simulink model "Lab2_EEN155_BUCK_2023"  (R2022b)
settings: Solver=VariableStepAuto  StartTime=0.0  StopTime=0.5  RelTol=1e-3
libraries: spsSeriesRLCBranchLib x4, spsCurrentMeasurementLib x4, spsVoltageMeasurementLib x3, spsDiodeLib x1, spsDCVoltageSourceLib x1, spsMosfetLib x1, spspowerguiLib x1
settings Model: Creator=emmag  LastModifiedBy=abdul
settings DebuggingCC: UnconnectedInputMsg=warning  UnconnectedOutputMsg=warning  UnconnectedLineMsg=warning
settings ModelReferenceCC: EnableRefExpFcnMdlSchedulingChecks=on
settings RTWCC: DLArmComputeVersion=19.05

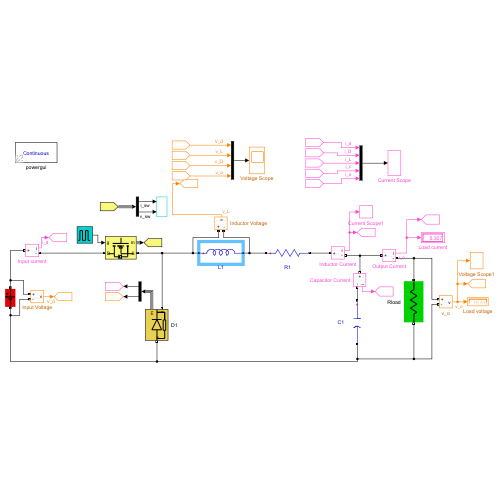
[thumbnail: Simulink's stored preview of the top-level diagram]
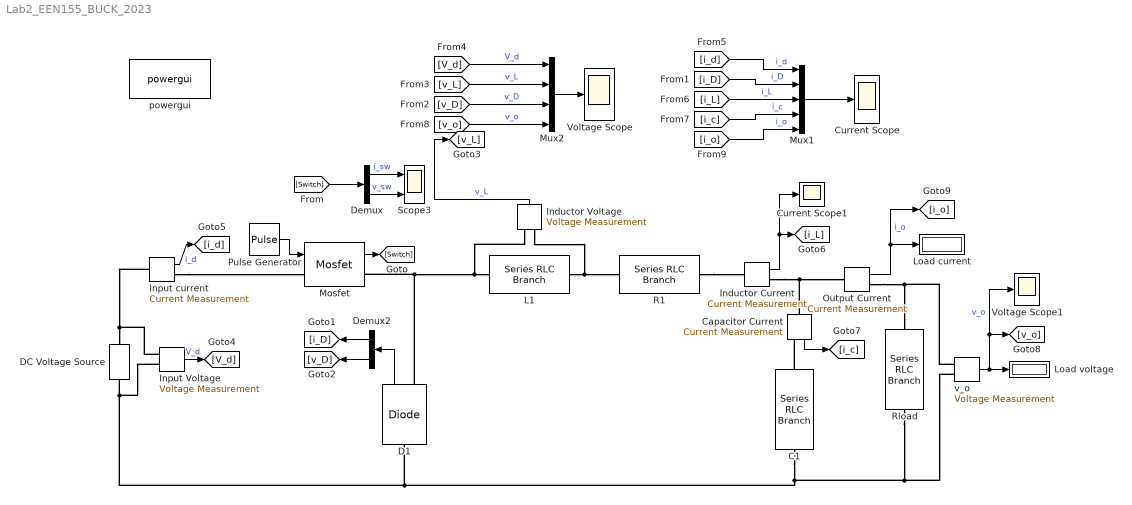
== system Lab2_EEN155_BUCK_2023 ==
  C1 : spsSeriesRLCBranchLib/Series RLC Branch  LConnTagsString=__new0  RConnTagsString=__new0  BranchType=C  Resistance=1  Inductance=1e-3  SetiL0=off  InitialCurrent=0  Capacitance=63e-6  Setx0=off  InitialVoltage=0  Measurements=None
  Capacitor Current : spsCurrentMeasurementLib/Current Measurement  PhasorSimulation=off  OutputType=Complex  PSBequivalent=0
  Current Scope : Scope
  Current Scope1 : Scope
  D1 : spsDiodeLib/Diode  Ron=0.001  Lon=0  Vf=0.8  IC=0  UseSnubber=0  Rs=500  Cs=250e-9  Measurements=on
  DC Voltage Source : spsDCVoltageSourceLib/DC Voltage Source  Amplitude=15  Measurements=None
  Demux : Demux  Outputs=2
  Demux2 : Demux  Outputs=2
  Inductor Current : spsCurrentMeasurementLib/Current Measurement  PhasorSimulation=off  OutputType=Complex  PSBequivalent=0
  Inductor Voltage : spsVoltageMeasurementLib/Voltage Measurement  PhasorSimulation=off  OutputType=Complex  PSBequivalent=0
  Input Voltage : spsVoltageMeasurementLib/Voltage Measurement  PhasorSimulation=off  OutputType=Complex  PSBequivalent=0
  Input current : spsCurrentMeasurementLib/Current Measurement  PhasorSimulation=off  OutputType=Complex  PSBequivalent=0
  L1 : spsSeriesRLCBranchLib/Series RLC Branch  LConnTagsString=__new0  RConnTagsString=__new0  BranchType=L  Resistance=1  Inductance=0.00025  SetiL0=off  InitialCurrent=0  Capacitance=1e-6  Setx0=off  InitialVoltage=0  Measurements=None
  Load current : Display
  Load voltage : Display
  Mosfet : spsMosfetLib/Mosfet  Ron=0.1  Lon=0  Rd=0.01  Vfd=0  IC=0  Rs=1e5  Cs=inf  Measurements=on
  Mux1 : Mux  Inputs=5
  Mux2 : Mux
  Output Current : spsCurrentMeasurementLib/Current Measurement  PhasorSimulation=off  OutputType=Complex  PSBequivalent=0
  Pulse Generator : DiscretePulseGenerator  PulseType=Time based  Period=1/20e3  PulseWidth=75
  R1 : spsSeriesRLCBranchLib/Series RLC Branch  LConnTagsString=__new0  RConnTagsString=__new0  BranchType=R  Resistance=10e-3  Inductance=1e-3  SetiL0=off  InitialCurrent=0  Capacitance=1e-6  Setx0=off  InitialVoltage=0  Measurements=None
  Rload : spsSeriesRLCBranchLib/Series RLC Branch  LConnTagsString=__new0  RConnTagsString=__new0  BranchType=R  Resistance=2  Inductance=1e-3  SetiL0=off  InitialCurrent=0  Capacitance=1e-6  Setx0=off  InitialVoltage=0  Measurements=None
  Scope3 : Scope  NumInputPorts=2
  Voltage Scope : Scope
  Voltage Scope1 : Scope
  powergui : spspowerguiLib/powergui  Priority=1  SimulationMode=Continuous  SampleTime=50e-6  frequency=60  Iterations=50  frequencyindice=0  Pbase=100e6  ErrMax=1e-4  UnitsV=kV  UnitsW=MW  buscounter=0  FunctionMessages=off  echomessages=off  EnableUseOfTLC=off  CurrentSourceSwitches=off  DisableSnubberDevices=off  DisableRonSwitches=off  DisableVfSwitches=off  DisplayEquations=off  AutomaticDiscreteSolvers=off  SolverType=Tustin/Backward Euler (TBE)  Interpol=off  ExternalGateDelay=off  methode=off  Ts=100  x0status=blocks  SPID=on  SwTol=0  HookPort=off  NonlinearTolerance=1e-4  nMaxIteration=100  ContinueOnMaxIteration=off  RestoreLinks=warning  ResistiveCurrentMeasurement=off  Frange=[0:2:500]  Ylog=off  Xlog=on  ShowGrid=off  save=off  variable=ZData  structure=0  ZoomFFT=off  StartTime=0.0  cycles=1  DisplayStyle=1  fundamental=60  FreqAxis=off  MaxFrequency=1000  frequencyindicesteady=1  RmsSteady=1  display=off
  v_o : spsVoltageMeasurementLib/Voltage Measurement  PhasorSimulation=off  OutputType=Complex  PSBequivalent=0
  wires:
  Pulse Generator/1 -> Mosfet/1
  v_o/1 -> Voltage Scope1/1, [v_o], Load voltage/1  "v_o"
  Output Current/1 -> [i_o], Load current/1  "i_o"
  Mux2/1 -> Voltage Scope/1
  Demux/1 -> Scope3/1  "i_sw"
  Demux/2 -> Scope3/2  "v_sw"
  Mosfet/1 -> [Switch]
  [Switch] -> Demux/1
  [i_D] -> Mux1/2  "i_D"
  [v_D] -> Mux2/3  "v_D"
  Mux1/1 -> Current Scope/1
  D1/1 -> Demux2/1
  Demux2/1 -> [i_D]
  Demux2/2 -> [v_D]
  Inductor Voltage/1 -> [v_L]  "v_L"
  Input Voltage/1 -> [V_d]  "V_d"
  [V_d] -> Mux2/1  "V_d"
  [v_L] -> Mux2/2  "v_L"
  Input current/1 -> [i_d]  "i_d"
  Capacitor Current/1 -> [i_c]
  [i_d] -> Mux1/1  "i_d"
  [i_L] -> Mux1/3  "i_L"
  [i_c] -> Mux1/4  "i_c"
  Inductor Current/1 -> [i_L], Current Scope1/1
  [v_o] -> Mux2/4  "v_o"
  [i_o] -> Mux1/5  "i_o"
  connections:
  D1/RConn1 -- Mosfet/RConn1 -- L1/LConn1 -- Inductor Voltage/LConn1
  L1/RConn1 -- R1/LConn1 -- Inductor Voltage/LConn2
  Inductor Current/RConn1 -- Capacitor Current/LConn1 -- Output Current/LConn1
  Output Current/RConn1 -- v_o/LConn1 -- Rload/LConn1
  D1/LConn1 -- Rload/RConn1 -- v_o/LConn2 -- C1/RConn1 -- Input Voltage/LConn2 -- DC Voltage Source/LConn1
  R1/RConn1 -- Inductor Current/LConn1
  C1/LConn1 -- Capacitor Current/RConn1
  Input current/RConn1 -- Mosfet/LConn1
  Input current/LConn1 -- Input Voltage/LConn1 -- DC Voltage Source/RConn1
